simulink model "simulate_robot_and_controller_line"  (Simulink 7.7)
settings: Solver=ode3  StartTime=0.0  StopTime=0.5  FixedStep=0.001  MaxStep=0.001  MinStep=0.0005  RelTol=1e-3
undefined symbols (not defined in the file or in its folder): call_direct_dynamics, robot
libraries: simulink x6
settings Model: Creator=arturo  LastModifiedBy=arturogilaparicio
settings DebuggingCC: StrictBusMsg=Warning

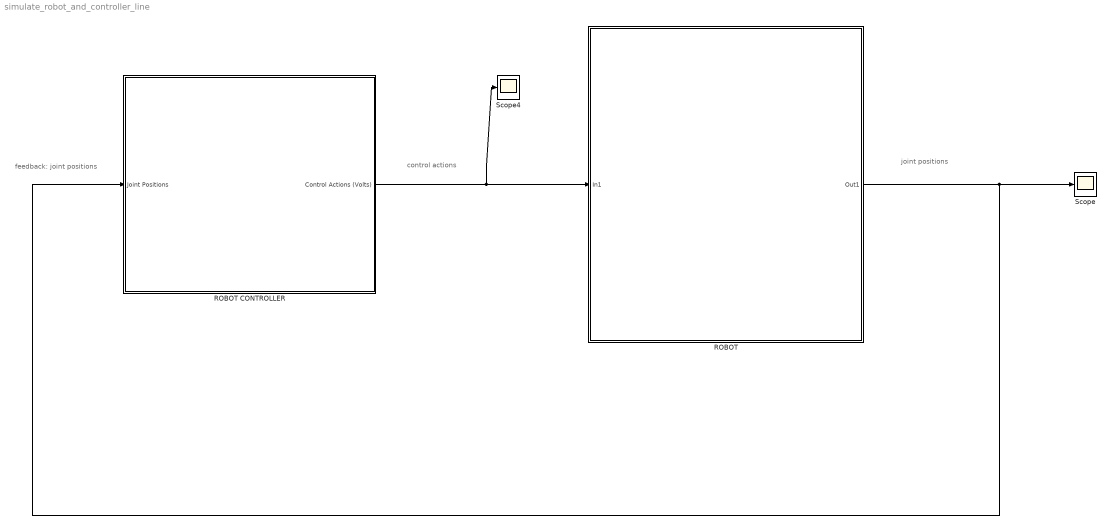
== system simulate_robot_and_controller_line ==
  note: control actions
  note: feedback: joint positions
  note: joint positions
  ROBOT : Subsystem
      mask Display:
      | port_label('output', 1, 'Joint positions (rad)')
      | port_label('input', 1, 'Control actions (Volts)')
      | image(imread('images/robot.png'))
  ROBOT CONTROLLER : Subsystem  Description=ROBOT CONTROLLER
      mask Display:
      | port_label('output', 1, 'Control Actions')
      | port_label('input', 1, 'Joint Positions')
      | image(imread('images/robot-controller.jpg'))
  Scope : Scope
      settings: TimeRange=0.5  YMin=-0.25  YMax=0.35
  Scope4 : Scope
      settings: YMin=-2.5  YMax=50  SaveName=ScopeData4
  wires:
  ROBOT CONTROLLER/1(Control Actions (Volts)) -> ROBOT/1(In1), Scope4/1
  ROBOT/1(Out1) -> ROBOT CONTROLLER/1(Joint Positions), Scope/1

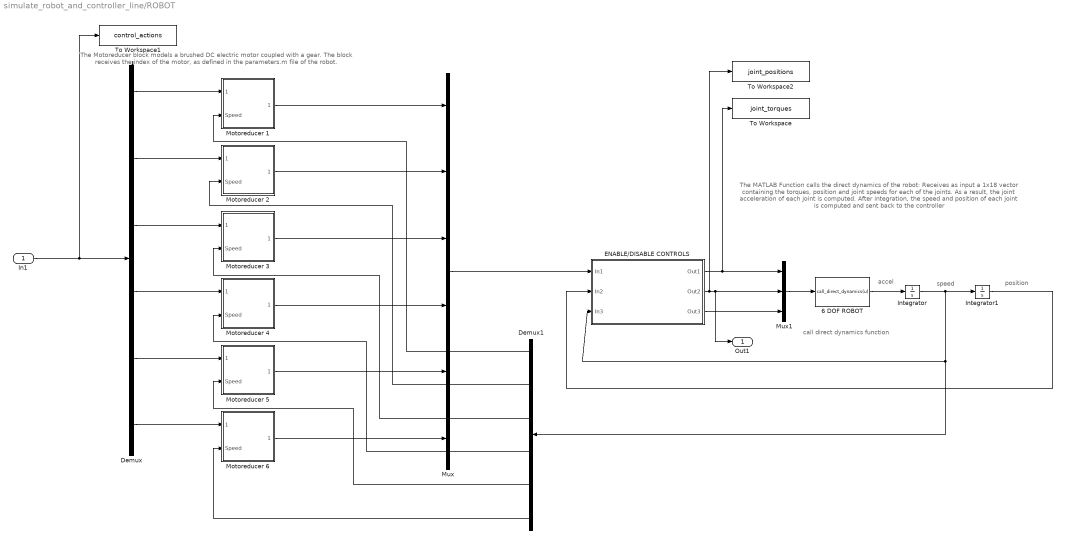
== system simulate_robot_and_controller_line/ROBOT ==
  note: accel
  note: speed
  note: position
  note: The MATLAB Function calls the direct dynamics of the robot:
      | Receives as input a 1x18 vector containing the
      | torques, position and joint
      | speeds for each of the joints. As a result, the joint
      | acceleration of each joint is computed.
      | After integration, the speed and position of each joint
      | is computed and sent back to the controller
  note: call direct dynamics
      |  function
  note: The Motoreducer block models a brushed DC
      | electric motor coupled with a gear.
      | The block receives the index of the motor,
      | as defined in the parameters.m file of the robot.
  In1 : Inport
  6 DOF ROBOT : MATLABFcn  MATLABFcn=call_direct_dynamics(u)  OutputDimensions=6
  Demux : Demux  Outputs=6
  Demux1 : Demux  Outputs=6
  ENABLE/DISABLE CONTROLS : Subsystem  mask{on_off_vector=[1 1 1 1 1 1]}
      mask prompts: on_off_vector "Set [1 1 1 1 1 1] to enable all motors and controls. Set [1 0 0 0 0 0] to enable just joint 1 control, [0 1 0 0 0 0] to enable 2, and so on:"
      mask Display:
      | port_label('input', 1, 'input_torque')
      | port_label('output', 1, 'output_torque')
      | port_label('input', 2, 'input_pos')
      | port_label('output', 2, 'output_pos')
      | port_label('input', 3, 'input_vel')
      | port_label('output', 3, 'output_vel')
  Integrator : Integrator  InitialCondition=[0 0 0 0 0 0]
  Integrator1 : Integrator  InitialCondition=[0 0 0 0 0.1 0]
  Motoreducer 1 : Subsystem  mask{index=1}
      mask prompts: index "Select motor index"
      mask Display: image(imread('images/brushless_dc.jpg'))
  Motoreducer 2 : Subsystem  mask{index=1}
      mask prompts: index "Select motor index"
      mask Display: image(imread('images/brushless_dc.jpg'))
  Motoreducer 3 : Subsystem  mask{index=1}
      mask prompts: index "Select motor index"
      mask Display: image(imread('images/brushless_dc.jpg'))
  Motoreducer 4 : Subsystem  mask{index=1}
      mask prompts: index "Select motor index"
      mask Display: image(imread('images/brushless_dc.jpg'))
  Motoreducer 5 : Subsystem  mask{index=1}
      mask prompts: index "Select motor index"
      mask Display: image(imread('images/brushless_dc.jpg'))
  Motoreducer 6 : Subsystem  mask{index=1}
      mask prompts: index "Select motor index"
      mask Display: image(imread('images/brushless_dc.jpg'))
  Mux : Mux  Inputs=6
  Mux1 : Mux  Inputs=3
  To Workspace : ToWorkspace  VariableName=joint_torques  SampleTime=-1  SaveFormat=Array
  To Workspace1 : ToWorkspace  VariableName=control_actions  SampleTime=-1  SaveFormat=Array
  To Workspace2 : ToWorkspace  VariableName=joint_positions  SampleTime=-1  SaveFormat=Array
  Out1 : Outport
  wires:
  Demux/1 -> Motoreducer 1/1(Input (Volts))
  Demux/2 -> Motoreducer 2/1(Input (Volts))
  Demux/3 -> Motoreducer 3/1(Input (Volts))
  Demux/5 -> Motoreducer 5/1(Input (Volts))
  Demux/6 -> Motoreducer 6/1(Input (Volts))
  Mux1/1 -> 6 DOF ROBOT/1
  6 DOF ROBOT/1 -> Integrator/1
  Integrator/1 -> Integrator1/1, ENABLE/DISABLE CONTROLS/3(In3), Demux1/1
  Mux/1 -> ENABLE/DISABLE CONTROLS/1(In1)
  Motoreducer 1/1(Output Torque) -> Mux/1
  Demux1/1 -> Motoreducer 1/2(Speed)
  Motoreducer 2/1(Output Torque) -> Mux/2
  Motoreducer 3/1(Output Torque) -> Mux/3
  Demux1/2 -> Motoreducer 2/2(Speed)
  Demux1/3 -> Motoreducer 3/2(Speed)
  Demux1/4 -> Motoreducer 4/2(Speed)
  Demux1/5 -> Motoreducer 5/2(Speed)
  Demux1/6 -> Motoreducer 6/2(Speed)
  Motoreducer 4/1(Output Torque) -> Mux/4
  Motoreducer 5/1(Output Torque) -> Mux/5
  Motoreducer 6/1(Output Torque) -> Mux/6
  In1/1 -> Demux/1, To Workspace1/1
  ENABLE/DISABLE CONTROLS/1(Out1) -> Mux1/1, To Workspace/1
  Demux/4 -> Motoreducer 4/1(Input (Volts))
  Integrator1/1 -> ENABLE/DISABLE CONTROLS/2(In2)
  ENABLE/DISABLE CONTROLS/2(Out2) -> Mux1/2, Out1/1, To Workspace2/1
  ENABLE/DISABLE CONTROLS/3(Out3) -> Mux1/3

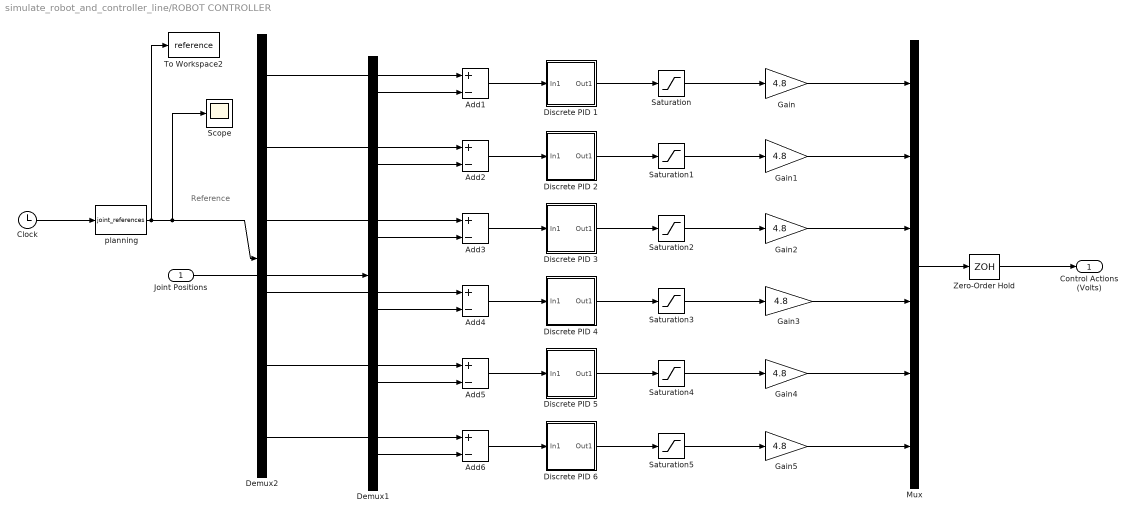
== system simulate_robot_and_controller_line/ROBOT CONTROLLER ==
  note: Reference
  Joint Positions : Inport  PortDimensions=6
  Add{1..6} (6 alike) : Sum  Inputs=+-
  Clock : Clock
      settings: Decimation=10
  Demux1 : Demux  Outputs=6
  Demux2 : Demux  Outputs=6
  Discrete PID 1 : Subsystem  mask{Kp=600, Kd=6, Ki=0, Ts=0.001}
      mask prompts: Kp "Proportional gain:"; Kd "Derivative gain:"; Ki "Integral gain:"; Ts "Sample time:"
      mask Display:
      | port_label('input',1,'e(k)')
      | port_label('output',1,'u(k)')
  Discrete PID 2 : Subsystem  mask{Kp=1000, Kd=10, Ki=5, Ts=0.001}
      mask prompts: Kp "Proportional gain:"; Kd "Derivative gain:"; Ki "Integral gain:"; Ts "Sample time:"
      mask Display:
      | port_label('input',1,'e(k)')
      | port_label('output',1,'u(k)')
  Discrete PID 3 : Subsystem  mask{Kp=800, Kd=7, Ki=5, Ts=0.001}
      mask prompts: Kp "Proportional gain:"; Kd "Derivative gain:"; Ki "Integral gain:"; Ts "Sample time:"
      mask Display:
      | port_label('input',1,'e(k)')
      | port_label('output',1,'u(k)')
  Discrete PID 4 : Subsystem  mask{Kp=2000, Kd=10, Ki=0, Ts=0.001}
      mask prompts: Kp "Proportional gain:"; Kd "Derivative gain:"; Ki "Integral gain:"; Ts "Sample time:"
      mask Display:
      | port_label('input',1,'e(k)')
      | port_label('output',1,'u(k)')
  Discrete PID 5 : Subsystem  mask{Kp=3000, Kd=7, Ki=3, Ts=0.001}
      mask prompts: Kp "Proportional gain:"; Kd "Derivative gain:"; Ki "Integral gain:"; Ts "Sample time:"
      mask Display:
      | port_label('input',1,'e(k)')
      | port_label('output',1,'u(k)')
  Discrete PID 6 : Subsystem  mask{Kp=3000, Kd=5, Ki=0, Ts=0.001}
      mask prompts: Kp "Proportional gain:"; Kd "Derivative gain:"; Ki "Integral gain:"; Ts "Sample time:"
      mask Display:
      | port_label('input',1,'e(k)')
      | port_label('output',1,'u(k)')
  Gain{,1..5} (6 alike) : Gain  Gain=4.8
  Mux : Mux  Inputs=6
  Saturation{,1..5} (6 alike) : Saturate  UpperLimit=10  LowerLimit=-10
  Scope : Scope
  To Workspace2 : ToWorkspace  VariableName=reference  SampleTime=-1  SaveFormat=Array
  Zero-Order Hold : ZeroOrderHold  SampleTime=0.001
  planning : MATLABFcn  MATLABFcn=joint_references  OutputDimensions=6
  Control Actions (Volts) : Outport
  wires:
  Gain5/1 -> Mux/6
  Gain4/1 -> Mux/5
  Gain3/1 -> Mux/4
  Gain2/1 -> Mux/3
  Gain1/1 -> Mux/2
  Gain/1 -> Mux/1
  Saturation5/1 -> Gain5/1
  Saturation4/1 -> Gain4/1
  Saturation3/1 -> Gain3/1
  Saturation2/1 -> Gain2/1
  Saturation1/1 -> Gain1/1
  Saturation/1 -> Gain/1
  Add6/1 -> Discrete PID 6/1(In1)
  Add5/1 -> Discrete PID 5/1(In1)
  Add4/1 -> Discrete PID 4/1(In1)
  Add3/1 -> Discrete PID 3/1(In1)
  Add2/1 -> Discrete PID 2/1(In1)
  Mux/1 -> Zero-Order Hold/1
  Joint Positions/1 -> Demux1/1
  Demux1/1 -> Add1/2
  Demux1/2 -> Add2/2
  Demux1/3 -> Add3/2
  Demux1/4 -> Add4/2
  Demux1/5 -> Add5/2
  Demux1/6 -> Add6/2
  Zero-Order Hold/1 -> Control Actions (Volts)/1
  Discrete PID 1/1(Out1) -> Saturation/1
  Add1/1 -> Discrete PID 1/1(In1)
  Discrete PID 2/1(Out1) -> Saturation1/1
  Discrete PID 3/1(Out1) -> Saturation2/1
  Discrete PID 4/1(Out1) -> Saturation3/1
  Discrete PID 5/1(Out1) -> Saturation4/1
  Discrete PID 6/1(Out1) -> Saturation5/1
  Clock/1 -> planning/1
  planning/1 -> To Workspace2/1, Demux2/1, Scope/1
  Demux2/1 -> Add1/1
  Demux2/2 -> Add2/1
  Demux2/3 -> Add3/1
  Demux2/4 -> Add4/1
  Demux2/5 -> Add5/1
  Demux2/6 -> Add6/1

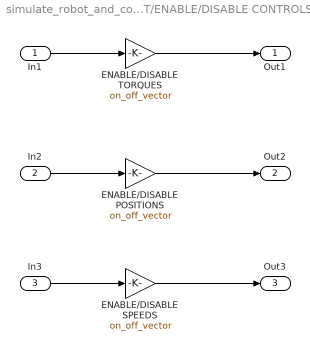
== system simulate_robot_and_controller_line/ROBOT/ENABLE/DISABLE CONTROLS ==
  In1 : Inport
  In2 : Inport  Port=2
  In3 : Inport  Port=3
  ENABLE/DISABLE POSITIONS : Gain  Gain=on_off_vector
  ENABLE/DISABLE SPEEDS : Gain  Gain=on_off_vector
  ENABLE/DISABLE TORQUES : Gain  Gain=on_off_vector
  Out1 : Outport
  Out2 : Outport  Port=2
  Out3 : Outport  Port=3
  wires:
  In2/1 -> ENABLE/DISABLE POSITIONS/1
  In1/1 -> ENABLE/DISABLE TORQUES/1
  ENABLE/DISABLE TORQUES/1 -> Out1/1
  In3/1 -> ENABLE/DISABLE SPEEDS/1
  ENABLE/DISABLE SPEEDS/1 -> Out3/1
  ENABLE/DISABLE POSITIONS/1 -> Out2/1

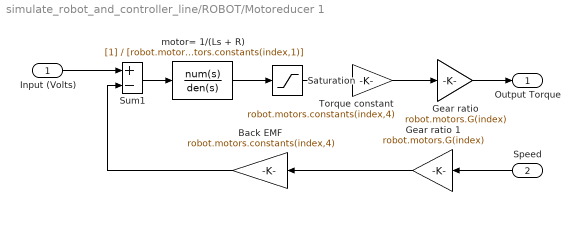
== system simulate_robot_and_controller_line/ROBOT/Motoreducer 1 ==
  Input (Volts) : Inport
  Speed : Inport  Port=2
  Back EMF : Gain  Gain=robot.motors.constants(index,4)  SaturateOnIntegerOverflow=on  OutDataTypeStr=Inherit: Same as input  ParamDataTypeStr=Inherit: Same as input
  Gear ratio : Gain  Gain=robot.motors.G(index)  SaturateOnIntegerOverflow=on  OutDataTypeStr=Inherit: Same as input  ParamDataTypeStr=Inherit: Same as input
  Gear ratio 1 : Gain  Gain=robot.motors.G(index)  SaturateOnIntegerOverflow=on  OutDataTypeStr=Inherit: Same as input  ParamDataTypeStr=Inherit: Same as input
  Saturation : Saturate  UpperLimit=robot.motors.constants(index,5)  LowerLimit=-robot.motors.constants(index,5)
  Sum1 : Sum  Inputs=+-  SaturateOnIntegerOverflow=on  InputSameDT=on  OutDataTypeStr=Inherit: Same as first input
  Torque constant : Gain  Gain=robot.motors.constants(index,4)  SaturateOnIntegerOverflow=on  OutDataTypeStr=Inherit: Same as input  ParamDataTypeStr=Inherit: Same as input
  motor= 1/(Ls + R) : TransferFcn  Denominator=[robot.motors.constants(index,2) robot.motors.constants(index,1)]
  Output Torque : Outport  InitialOutput=0
  wires:
  Saturation/1 -> Torque constant/1
  motor= 1/(Ls + R)/1 -> Saturation/1
  Torque constant/1 -> Gear ratio/1
  Gear ratio/1 -> Output Torque/1
  Sum1/1 -> motor= 1/(Ls + R)/1
  Gear ratio 1/1 -> Back EMF/1
  Back EMF/1 -> Sum1/2
  Input (Volts)/1 -> Sum1/1
  Speed/1 -> Gear ratio 1/1

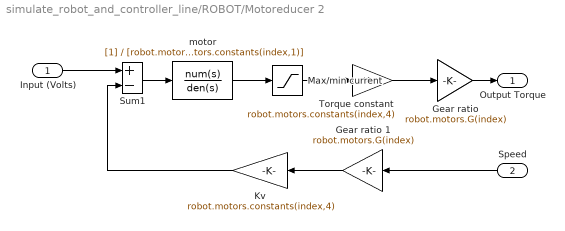
== system simulate_robot_and_controller_line/ROBOT/Motoreducer 2 ==
  Input (Volts) : Inport
  Speed : Inport  Port=2
  Gear ratio : Gain  Gain=robot.motors.G(index)  SaturateOnIntegerOverflow=on  OutDataTypeStr=Inherit: Same as input  ParamDataTypeStr=Inherit: Same as input
  Gear ratio 1 : Gain  Gain=robot.motors.G(index)  SaturateOnIntegerOverflow=on  OutDataTypeStr=Inherit: Same as input  ParamDataTypeStr=Inherit: Same as input
  Kv : Gain  Gain=robot.motors.constants(index,4)  SaturateOnIntegerOverflow=on  OutDataTypeStr=Inherit: Same as input  ParamDataTypeStr=Inherit: Same as input
  Max/min current : Saturate  UpperLimit=robot.motors.constants(index,5)  LowerLimit=-robot.motors.constants(index,5)
  Sum1 : Sum  Inputs=+-  SaturateOnIntegerOverflow=on  InputSameDT=on  OutDataTypeStr=Inherit: Same as first input
  Torque constant : Gain  Gain=robot.motors.constants(index,4)  SaturateOnIntegerOverflow=on  OutDataTypeStr=Inherit: Same as input  ParamDataTypeStr=Inherit: Same as input
  motor : TransferFcn  Denominator=[robot.motors.constants(index,2) robot.motors.constants(index,1)]
  Output Torque : Outport  InitialOutput=0
  wires:
  Max/min current/1 -> Torque constant/1
  motor/1 -> Max/min current/1
  Torque constant/1 -> Gear ratio/1
  Gear ratio/1 -> Output Torque/1
  Sum1/1 -> motor/1
  Gear ratio 1/1 -> Kv/1
  Kv/1 -> Sum1/2
  Input (Volts)/1 -> Sum1/1
  Speed/1 -> Gear ratio 1/1

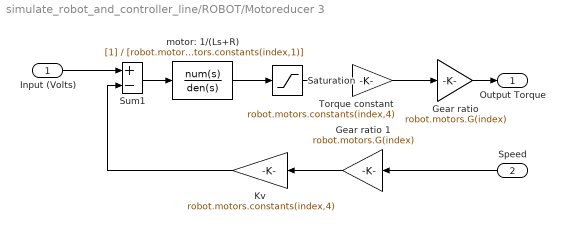
== system simulate_robot_and_controller_line/ROBOT/Motoreducer 3 ==
  Input (Volts) : Inport
  Speed : Inport  Port=2
  Gear ratio : Gain  Gain=robot.motors.G(index)  SaturateOnIntegerOverflow=on  OutDataTypeStr=Inherit: Same as input  ParamDataTypeStr=Inherit: Same as input
  Gear ratio 1 : Gain  Gain=robot.motors.G(index)  SaturateOnIntegerOverflow=on  OutDataTypeStr=Inherit: Same as input  ParamDataTypeStr=Inherit: Same as input
  Kv : Gain  Gain=robot.motors.constants(index,4)  SaturateOnIntegerOverflow=on  OutDataTypeStr=Inherit: Same as input  ParamDataTypeStr=Inherit: Same as input
  Saturation : Saturate  UpperLimit=robot.motors.constants(index,5)  LowerLimit=-robot.motors.constants(index,5)
  Sum1 : Sum  Inputs=+-  SaturateOnIntegerOverflow=on  InputSameDT=on  OutDataTypeStr=Inherit: Same as first input
  Torque constant : Gain  Gain=robot.motors.constants(index,4)  SaturateOnIntegerOverflow=on  OutDataTypeStr=Inherit: Same as input  ParamDataTypeStr=Inherit: Same as input
  motor: 1/(Ls+R) : TransferFcn  Denominator=[robot.motors.constants(index,2) robot.motors.constants(index,1)]
  Output Torque : Outport  InitialOutput=0
  wires:
  Saturation/1 -> Torque constant/1
  motor: 1/(Ls+R)/1 -> Saturation/1
  Torque constant/1 -> Gear ratio/1
  Gear ratio/1 -> Output Torque/1
  Sum1/1 -> motor: 1/(Ls+R)/1
  Gear ratio 1/1 -> Kv/1
  Kv/1 -> Sum1/2
  Input (Volts)/1 -> Sum1/1
  Speed/1 -> Gear ratio 1/1

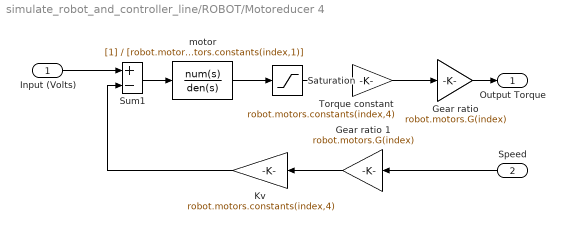
== system simulate_robot_and_controller_line/ROBOT/Motoreducer 4 ==
  Input (Volts) : Inport
  Speed : Inport  Port=2
  Gear ratio : Gain  Gain=robot.motors.G(index)  SaturateOnIntegerOverflow=on  OutDataTypeStr=Inherit: Same as input  ParamDataTypeStr=Inherit: Same as input
  Gear ratio 1 : Gain  Gain=robot.motors.G(index)  SaturateOnIntegerOverflow=on  OutDataTypeStr=Inherit: Same as input  ParamDataTypeStr=Inherit: Same as input
  Kv : Gain  Gain=robot.motors.constants(index,4)  SaturateOnIntegerOverflow=on  OutDataTypeStr=Inherit: Same as input  ParamDataTypeStr=Inherit: Same as input
  Saturation : Saturate  UpperLimit=robot.motors.constants(index,5)  LowerLimit=-robot.motors.constants(index,5)
  Sum1 : Sum  Inputs=+-  SaturateOnIntegerOverflow=on  InputSameDT=on  OutDataTypeStr=Inherit: Same as first input
  Torque constant : Gain  Gain=robot.motors.constants(index,4)  SaturateOnIntegerOverflow=on  OutDataTypeStr=Inherit: Same as input  ParamDataTypeStr=Inherit: Same as input
  motor : TransferFcn  Denominator=[robot.motors.constants(index,2) robot.motors.constants(index,1)]
  Output Torque : Outport  InitialOutput=0
  wires:
  Saturation/1 -> Torque constant/1
  motor/1 -> Saturation/1
  Torque constant/1 -> Gear ratio/1
  Gear ratio/1 -> Output Torque/1
  Sum1/1 -> motor/1
  Gear ratio 1/1 -> Kv/1
  Kv/1 -> Sum1/2
  Input (Volts)/1 -> Sum1/1
  Speed/1 -> Gear ratio 1/1

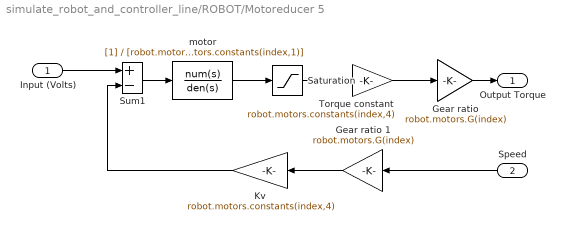
== system simulate_robot_and_controller_line/ROBOT/Motoreducer 5 ==
  Input (Volts) : Inport
  Speed : Inport  Port=2
  Gear ratio : Gain  Gain=robot.motors.G(index)  SaturateOnIntegerOverflow=on  OutDataTypeStr=Inherit: Same as input  ParamDataTypeStr=Inherit: Same as input
  Gear ratio 1 : Gain  Gain=robot.motors.G(index)  SaturateOnIntegerOverflow=on  OutDataTypeStr=Inherit: Same as input  ParamDataTypeStr=Inherit: Same as input
  Kv : Gain  Gain=robot.motors.constants(index,4)  SaturateOnIntegerOverflow=on  OutDataTypeStr=Inherit: Same as input  ParamDataTypeStr=Inherit: Same as input
  Saturation : Saturate  UpperLimit=robot.motors.constants(index,5)  LowerLimit=-robot.motors.constants(index,5)
  Sum1 : Sum  Inputs=+-  SaturateOnIntegerOverflow=on  InputSameDT=on  OutDataTypeStr=Inherit: Same as first input
  Torque constant : Gain  Gain=robot.motors.constants(index,4)  SaturateOnIntegerOverflow=on  OutDataTypeStr=Inherit: Same as input  ParamDataTypeStr=Inherit: Same as input
  motor : TransferFcn  Denominator=[robot.motors.constants(index,2) robot.motors.constants(index,1)]
  Output Torque : Outport  InitialOutput=0
  wires:
  Saturation/1 -> Torque constant/1
  motor/1 -> Saturation/1
  Torque constant/1 -> Gear ratio/1
  Gear ratio/1 -> Output Torque/1
  Sum1/1 -> motor/1
  Gear ratio 1/1 -> Kv/1
  Kv/1 -> Sum1/2
  Input (Volts)/1 -> Sum1/1
  Speed/1 -> Gear ratio 1/1

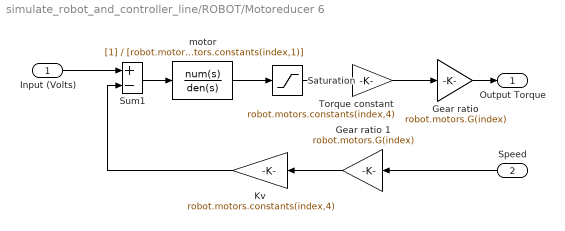
== system simulate_robot_and_controller_line/ROBOT/Motoreducer 6 ==
  Input (Volts) : Inport
  Speed : Inport  Port=2
  Gear ratio : Gain  Gain=robot.motors.G(index)  SaturateOnIntegerOverflow=on  OutDataTypeStr=Inherit: Same as input  ParamDataTypeStr=Inherit: Same as input
  Gear ratio 1 : Gain  Gain=robot.motors.G(index)  SaturateOnIntegerOverflow=on  OutDataTypeStr=Inherit: Same as input  ParamDataTypeStr=Inherit: Same as input
  Kv : Gain  Gain=robot.motors.constants(index,4)  SaturateOnIntegerOverflow=on  OutDataTypeStr=Inherit: Same as input  ParamDataTypeStr=Inherit: Same as input
  Saturation : Saturate  UpperLimit=robot.motors.constants(index,5)  LowerLimit=-robot.motors.constants(index,5)
  Sum1 : Sum  Inputs=+-  SaturateOnIntegerOverflow=on  InputSameDT=on  OutDataTypeStr=Inherit: Same as first input
  Torque constant : Gain  Gain=robot.motors.constants(index,4)  SaturateOnIntegerOverflow=on  OutDataTypeStr=Inherit: Same as input  ParamDataTypeStr=Inherit: Same as input
  motor : TransferFcn  Denominator=[robot.motors.constants(index,2) robot.motors.constants(index,1)]
  Output Torque : Outport  InitialOutput=0
  wires:
  Saturation/1 -> Torque constant/1
  motor/1 -> Saturation/1
  Torque constant/1 -> Gear ratio/1
  Gear ratio/1 -> Output Torque/1
  Sum1/1 -> motor/1
  Gear ratio 1/1 -> Kv/1
  Kv/1 -> Sum1/2
  Input (Volts)/1 -> Sum1/1
  Speed/1 -> Gear ratio 1/1

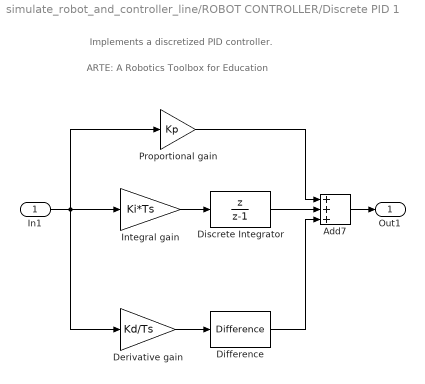
== system simulate_robot_and_controller_line/ROBOT CONTROLLER/Discrete PID 1 ==
  note: Implements a discretized PID controller.
  note: ARTE: A Robotics Toolbox for Education
  In1 : Inport
  Add7 : Sum  Inputs=+++
  Derivative gain : Gain  Gain=Kd/Ts
  Difference : simulink/Discrete/Difference  SystemSampleTime=-1  ICPrevInput=0.0  OutMin=[]  OutMax=[]  OutDataType=fixdt(1, 16)  OutScaling=2^-10  DoSatur=off
  Discrete Integrator : DiscreteTransferFcn  Numerator=[1 0]  Denominator=[1 -1]  SampleTime=Ts
  Integral gain : Gain  Gain=Ki*Ts
  Proportional gain : Gain  Gain=Kp
  Out1 : Outport
  wires:
  In1/1 -> Derivative gain/1, Proportional gain/1, Integral gain/1
  Discrete Integrator/1 -> Add7/2
  Difference/1 -> Add7/3
  Integral gain/1 -> Discrete Integrator/1
  Derivative gain/1 -> Difference/1
  Proportional gain/1 -> Add7/1
  Add7/1 -> Out1/1

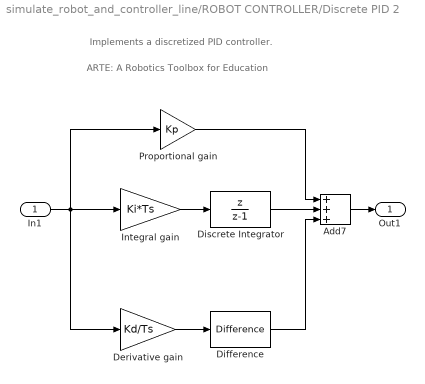
== system simulate_robot_and_controller_line/ROBOT CONTROLLER/Discrete PID 2 ==
  note: Implements a discretized PID controller.
  note: ARTE: A Robotics Toolbox for Education
  In1 : Inport
  Add7 : Sum  Inputs=+++
  Derivative gain : Gain  Gain=Kd/Ts
  Difference : simulink/Discrete/Difference  SystemSampleTime=-1  ICPrevInput=0.0  OutMin=[]  OutMax=[]  OutDataType=fixdt(1, 16)  OutScaling=2^-10  DoSatur=off
  Discrete Integrator : DiscreteTransferFcn  Numerator=[1 0]  Denominator=[1 -1]  SampleTime=Ts
  Integral gain : Gain  Gain=Ki*Ts
  Proportional gain : Gain  Gain=Kp
  Out1 : Outport
  wires:
  In1/1 -> Derivative gain/1, Proportional gain/1, Integral gain/1
  Discrete Integrator/1 -> Add7/2
  Difference/1 -> Add7/3
  Integral gain/1 -> Discrete Integrator/1
  Derivative gain/1 -> Difference/1
  Proportional gain/1 -> Add7/1
  Add7/1 -> Out1/1

== system simulate_robot_and_controller_line/ROBOT CONTROLLER/Discrete PID 3 ==
  note: Implements a discretized PID controller.
  note: ARTE: A Robotics Toolbox for Education
  In1 : Inport
  Add7 : Sum  Inputs=+++
  Derivative gain : Gain  Gain=Kd/Ts
  Difference : simulink/Discrete/Difference  SystemSampleTime=-1  ICPrevInput=0.0  OutMin=[]  OutMax=[]  OutDataType=fixdt(1, 16)  OutScaling=2^-10  DoSatur=off
  Discrete Integrator : DiscreteTransferFcn  Numerator=[1 0]  Denominator=[1 -1]  SampleTime=Ts
  Integral gain : Gain  Gain=Ki*Ts
  Proportional gain : Gain  Gain=Kp
  Out1 : Outport
  wires:
  In1/1 -> Derivative gain/1, Proportional gain/1, Integral gain/1
  Discrete Integrator/1 -> Add7/2
  Difference/1 -> Add7/3
  Integral gain/1 -> Discrete Integrator/1
  Derivative gain/1 -> Difference/1
  Proportional gain/1 -> Add7/1
  Add7/1 -> Out1/1

== system simulate_robot_and_controller_line/ROBOT CONTROLLER/Discrete PID 4 ==
  note: Implements a discretized PID controller.
  note: ARTE: A Robotics Toolbox for Education
  In1 : Inport
  Add7 : Sum  Inputs=+++
  Derivative gain : Gain  Gain=Kd/Ts
  Difference : simulink/Discrete/Difference  SystemSampleTime=-1  ICPrevInput=0.0  OutMin=[]  OutMax=[]  OutDataType=fixdt(1, 16)  OutScaling=2^-10  DoSatur=off
  Discrete Integrator : DiscreteTransferFcn  Numerator=[1 0]  Denominator=[1 -1]  SampleTime=Ts
  Integral gain : Gain  Gain=Ki*Ts
  Proportional gain : Gain  Gain=Kp
  Out1 : Outport
  wires:
  In1/1 -> Derivative gain/1, Proportional gain/1, Integral gain/1
  Discrete Integrator/1 -> Add7/2
  Difference/1 -> Add7/3
  Integral gain/1 -> Discrete Integrator/1
  Derivative gain/1 -> Difference/1
  Proportional gain/1 -> Add7/1
  Add7/1 -> Out1/1

== system simulate_robot_and_controller_line/ROBOT CONTROLLER/Discrete PID 5 ==
  note: Implements a discretized PID controller.
  note: ARTE: A Robotics Toolbox for Education
  In1 : Inport
  Add7 : Sum  Inputs=+++
  Derivative gain : Gain  Gain=Kd/Ts
  Difference : simulink/Discrete/Difference  SystemSampleTime=-1  ICPrevInput=0.0  OutMin=[]  OutMax=[]  OutDataType=fixdt(1, 16)  OutScaling=2^-10  DoSatur=off
  Discrete Integrator : DiscreteTransferFcn  Numerator=[1 0]  Denominator=[1 -1]  SampleTime=Ts
  Integral gain : Gain  Gain=Ki*Ts
  Proportional gain : Gain  Gain=Kp
  Out1 : Outport
  wires:
  In1/1 -> Derivative gain/1, Proportional gain/1, Integral gain/1
  Discrete Integrator/1 -> Add7/2
  Difference/1 -> Add7/3
  Integral gain/1 -> Discrete Integrator/1
  Derivative gain/1 -> Difference/1
  Proportional gain/1 -> Add7/1
  Add7/1 -> Out1/1

== system simulate_robot_and_controller_line/ROBOT CONTROLLER/Discrete PID 6 ==
  note: Implements a discretized PID controller.
  note: ARTE: A Robotics Toolbox for Education
  In1 : Inport
  Add7 : Sum  Inputs=+++
  Derivative gain : Gain  Gain=Kd/Ts
  Difference : simulink/Discrete/Difference  SystemSampleTime=-1  ICPrevInput=0.0  OutMin=[]  OutMax=[]  OutDataType=fixdt(1, 16)  OutScaling=2^-10  DoSatur=off
  Discrete Integrator : DiscreteTransferFcn  Numerator=[1 0]  Denominator=[1 -1]  SampleTime=Ts
  Integral gain : Gain  Gain=Ki*Ts
  Proportional gain : Gain  Gain=Kp
  Out1 : Outport
  wires:
  In1/1 -> Derivative gain/1, Proportional gain/1, Integral gain/1
  Discrete Integrator/1 -> Add7/2
  Difference/1 -> Add7/3
  Integral gain/1 -> Discrete Integrator/1
  Derivative gain/1 -> Difference/1
  Proportional gain/1 -> Add7/1
  Add7/1 -> Out1/1
